simulink library "dspmtrx3"  (Simulink 8.0)
settings: Solver=ode45  SolverMode=SingleTasking  StartTime=0.0  StopTime=10.0  RelTol=1e-3
values from neighbouring files (symbols this model uses):
  a = ver('dsp')    [aboutdspsystbx.m]    (also in dsparch3Transform.m = localGetVal(inData.InstanceData, 'den', '1'); dspddes3Transform.m = sprintf('getYuleWalkerIIRFilterDesignOutput(; dspfdes.m = []; dsprprim.m = a-Mi)
  D = D + B    [rebuffer_delay.m]
undefined symbols (not defined in the file or in its folder): Floor
libraries: dspmtrx3 x5, dspsolvers x3, dspsigattribs x2, dspobslib x1, dspstat3 x1, dspfactors x1
(part 2 of 2)

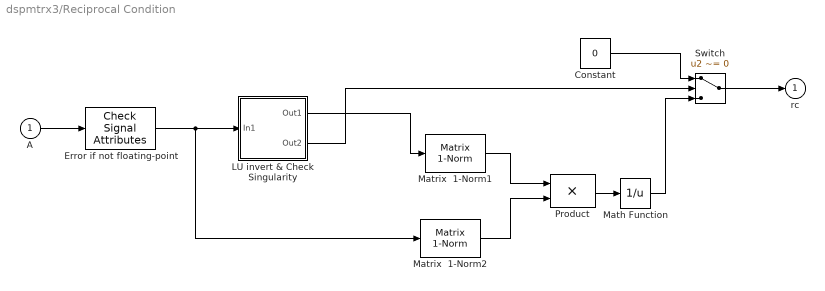
== system dspmtrx3/Reciprocal Condition ==
  A : Inport
  Constant : Constant  Value=0  OutDataTypeStr=Inherit: Inherit via back propagation
  Error if not floating-point : dspsigattribs/Check Signal Attributes  SystemSampleTime=-1  SigAttribCheckMethod=Does not match attributes exactly  Complexity=Ignore  Frame=Ignore  DimsCheckMethod=Ignore  Dimensions=1-D  DatatypeCheckMethod=Is...  DatatypeGeneral=Floating-point  DtypeFloatSpecific=Any floating-point  DtypeFixedSpecific=Any fixed-point  DtypeIntSpecific=Any integer  SampleMode=Ignore
  LU invert & Check Singularity : Subsystem
      mask Display:
      | port_label('output',1,'Inv');
      | port_label('output',2,'Status');
      | port_label('input',1,'Mx');
  Math Function : Math  Operator=reciprocal  SaturateOnIntegerOverflow=on
  Matrix  1-Norm1 : dspmtrx3/Matrix  1-Norm  outputDataTypeStr=Inherit: Same as accumulator  outputLastDataTypeStr=Inherit: Same as accumulator  outputMin=[]  outputMax=[]  roundingMode=Floor  overflowMode=off
  Matrix  1-Norm2 : dspmtrx3/Matrix  1-Norm  outputDataTypeStr=Inherit: Same as accumulator  outputLastDataTypeStr=Inherit: Same as accumulator  outputMin=[]  outputMax=[]  roundingMode=Floor  overflowMode=off
  Product : Product  SaturateOnIntegerOverflow=on  InputSameDT=on  OutDataTypeStr=Inherit: Same as first input
  Switch : Switch  Criteria=u2 ~= 0  InputSameDT=on
  " rc" : Outport  InitialOutput=0
  wires:
  LU invert & Check Singularity/2(Out2) -> Switch/2
  Math Function/1 -> Switch/3
  Switch/1 -> " rc"/1
  Product/1 -> Math Function/1
  Matrix  1-Norm2/1 -> Product/2
  Matrix  1-Norm1/1 -> Product/1
  Constant/1 -> Switch/1
  LU invert & Check Singularity/1(Out1) -> Matrix  1-Norm1/1
  A/1 -> Error if not floating-point/1
  Error if not floating-point/1 -> LU invert & Check Singularity/1(In1), Matrix  1-Norm2/1

== system dspmtrx3/Transpose ==
  In1 : Inport
  Math Function : Math  Operator=transpose  SaturateOnIntegerOverflow=on
  Out1 : Outport
  wires:
  In1/1 -> Math Function/1
  Math Function/1 -> Out1/1

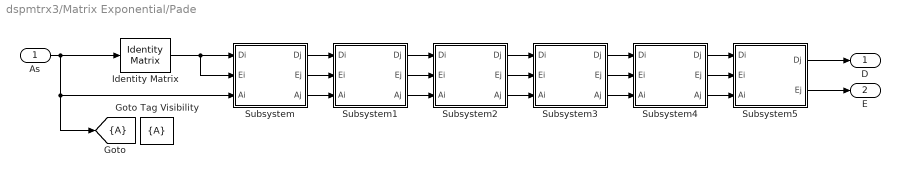
== system dspmtrx3/Matrix Exponential/Pade ==
  As : Inport
  Goto Tag Visibility : GotoTagVisibility
  Identity Matrix : dspmtrx3/Identity Matrix  Inherit=on  N=5  Ts=1  dataType=double  isSigned=on  wordLen=16  udDataType=sfix(16)  fracBitsMode=Best precision  numFracBits=15
  Subsystem : Subsystem
      mask Display: disp('Pade\n1')
  Subsystem1 : Subsystem
      mask Display: disp('Pade\n2')
  Subsystem2 : Subsystem
      mask Display: disp('Pade\n3')
  Subsystem3 : Subsystem
      mask Display: disp('Pade\n4')
  Subsystem4 : Subsystem
      mask Display: disp('Pade\n5')
  Subsystem5 : Subsystem
      mask Display: disp('Pade\n6')
  D : Outport
  E : Outport  Port=2
  tag scope: A=scoped
  wires:
  As/1 -> Identity Matrix/1, Subsystem/3(Ai), [A]
  Identity Matrix/1 -> Subsystem/1(Di), Subsystem/2(Ei)
  Subsystem/1(Dj) -> Subsystem1/1(Di)
  Subsystem/2(Ej) -> Subsystem1/2(Ei)
  Subsystem1/1(Dj) -> Subsystem2/1(Di)
  Subsystem1/2(Ej) -> Subsystem2/2(Ei)
  Subsystem2/1(Dj) -> Subsystem3/1(Di)
  Subsystem2/2(Ej) -> Subsystem3/2(Ei)
  Subsystem3/1(Dj) -> Subsystem4/1(Di)
  Subsystem3/2(Ej) -> Subsystem4/2(Ei)
  Subsystem4/1(Dj) -> Subsystem5/1(Di)
  Subsystem4/2(Ej) -> Subsystem5/2(Ei)
  Subsystem5/2(Ej) -> E/1
  Subsystem5/1(Dj) -> D/1
  Subsystem/3(Aj) -> Subsystem1/3(Ai)
  Subsystem1/3(Aj) -> Subsystem2/3(Ai)
  Subsystem2/3(Aj) -> Subsystem3/3(Ai)
  Subsystem3/3(Aj) -> Subsystem4/3(Ai)
  Subsystem4/3(Aj) -> Subsystem5/3(Ai)

== system dspmtrx3/Matrix Exponential/Scale In ==
  A : Inport
  Inf norm : Subsystem
      mask Display: disp('inf\nnorm')
  Pow2 Scaling : Subsystem
      mask Display: disp('s-scaling')
  Scale Input : Subsystem
  log2 : Subsystem
      mask Display: disp('log2')
  As : Outport
  s : Outport  Port=2
  wires:
  A/1 -> Inf norm/1(In1), Scale Input/2(A)
  Inf norm/1(Out1) -> log2/1(u)
  log2/1(e) -> Pow2 Scaling/1(In1)
  Pow2 Scaling/1(Out1) -> Scale Input/1(s), s/1
  Scale Input/1(sA) -> As/1

== system dspmtrx3/Matrix Exponential/Scale Out ==
  E : Inport
  s : Inport  Port=2
  Frame Conversion : FrameConversion  OutFrame=Sample-based
  Matrix Squaring : Subsystem  TreatAsAtomicUnit=on
  Switch : Switch  Criteria=u2 ~= 0  SaturateOnIntegerOverflow=on
  expm : Outport
  wires:
  s/1 -> Switch/2, Frame Conversion/1
  E/1 -> Matrix Squaring/1(E), Switch/3
  Matrix Squaring/1(Out) -> Switch/1
  Switch/1 -> expm/1
  Frame Conversion/1 -> Matrix Squaring/2(N)

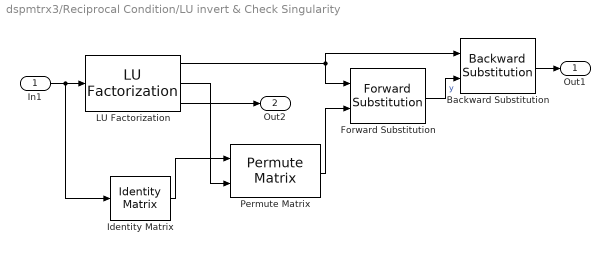
== system dspmtrx3/Reciprocal Condition/LU invert & Check Singularity ==
  In1 : Inport
  Backward Substitution : dspsolvers/Backward Substitution  Unit=off  RealDiag=off  outputMin=[]  outputMax=[]  accumDataTypeStr=Inherit: Same as product output  accumLastDataTypeStr=Inherit: Same as product output  roundingMode=Floor  overflowMode=off
  Forward Substitution : dspsolvers/Forward Substitution  Unit=on  RealDiag=on  outputMin=[]  outputMax=[]  accumDataTypeStr=Inherit: Same as product output  accumLastDataTypeStr=Inherit: Same as product output  roundingMode=Floor  overflowMode=off
  Identity Matrix : dspmtrx3/Identity Matrix  Inherit=on  N=5  Ts=1  dataType=double  isSigned=on  wordLen=16  udDataType=sfix(16)  fracBitsMode=Best precision  numFracBits=15
  LU Factorization : dspfactors/LU Factorization  singular=on  roundingMode=Floor  overflowMode=off
  Permute Matrix : dspmtrx3/Permute Matrix  mode=Rows  ZeroOneIdxMode=One-based  errmode=Clip index  checkDims=on
  Out1 : Outport
  Out2 : Outport  Port=2
  wires:
  LU Factorization/3 -> Out2/1
  LU Factorization/2 -> Permute Matrix/2
  LU Factorization/1 -> Backward Substitution/1, Forward Substitution/1
  Backward Substitution/1 -> Out1/1
  In1/1 -> LU Factorization/1, Identity Matrix/1
  Forward Substitution/1 -> Backward Substitution/2  "y"
  Permute Matrix/1 -> Forward Substitution/2
  Identity Matrix/1 -> Permute Matrix/1

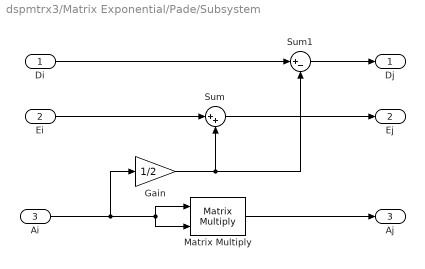
== system dspmtrx3/Matrix Exponential/Pade/Subsystem ==
  Di : Inport
  Ei : Inport  Port=2
  Ai : Inport  Port=3
  Gain : Gain  Gain=1/2  SaturateOnIntegerOverflow=on  OutDataTypeStr=Inherit: Same as input  ParamDataTypeStr=Inherit: Same as input
  Matrix Multiply : Product  Multiplication=Matrix(*)
  Sum : Sum  Inputs=|++  OutDataTypeStr=Inherit: Inherit via back propagation  SaturateOnIntegerOverflow=on
  Sum1 : Sum  Inputs=|+-  OutDataTypeStr=Inherit: Inherit via back propagation  SaturateOnIntegerOverflow=on
  Dj : Outport
  Ej : Outport  Port=2
  Aj : Outport  Port=3
  wires:
  Ei/1 -> Sum/1
  Sum/1 -> Ej/1
  Sum1/1 -> Dj/1
  Di/1 -> Sum1/1
  Gain/1 -> Sum/2, Sum1/2
  Ai/1 -> Gain/1, Matrix Multiply/2, Matrix Multiply/1
  Matrix Multiply/1 -> Aj/1

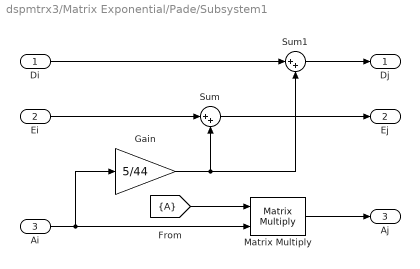
== system dspmtrx3/Matrix Exponential/Pade/Subsystem1 ==
  Di : Inport
  Ei : Inport  Port=2
  Ai : Inport  Port=3
  Gain : Gain  Gain=5/44  OutDataTypeStr=Inherit: Same as input  ParamDataTypeStr=Inherit: Same as input
  Matrix Multiply : Product  Multiplication=Matrix(*)
  Sum : Sum  Inputs=|++  OutDataTypeStr=Inherit: Inherit via back propagation  SaturateOnIntegerOverflow=on
  Sum1 : Sum  Inputs=|++  OutDataTypeStr=Inherit: Inherit via back propagation  SaturateOnIntegerOverflow=on
  Dj : Outport
  Ej : Outport  Port=2
  Aj : Outport  Port=3
  wires:
  Di/1 -> Sum1/1
  Sum1/1 -> Dj/1
  Sum/1 -> Ej/1
  Ei/1 -> Sum/1
  Gain/1 -> Sum/2, Sum1/2
  Ai/1 -> Gain/1, Matrix Multiply/2
  Matrix Multiply/1 -> Aj/1
  [A] -> Matrix Multiply/1

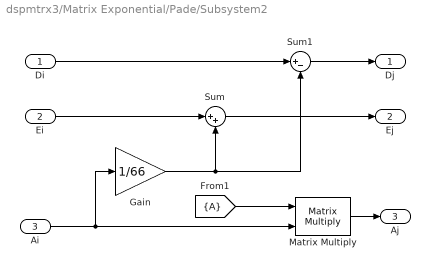
== system dspmtrx3/Matrix Exponential/Pade/Subsystem2 ==
  Di : Inport
  Ei : Inport  Port=2
  Ai : Inport  Port=3
  Gain : Gain  Gain=1/66  OutDataTypeStr=Inherit: Same as input  ParamDataTypeStr=Inherit: Same as input
  Matrix Multiply : Product  Multiplication=Matrix(*)
  Sum : Sum  Inputs=|++  OutDataTypeStr=Inherit: Inherit via back propagation  SaturateOnIntegerOverflow=on
  Sum1 : Sum  Inputs=|+-  OutDataTypeStr=Inherit: Inherit via back propagation  SaturateOnIntegerOverflow=on
  Dj : Outport
  Ej : Outport  Port=2
  Aj : Outport  Port=3
  wires:
  Gain/1 -> Sum1/2, Sum/2
  Di/1 -> Sum1/1
  Sum1/1 -> Dj/1
  Sum/1 -> Ej/1
  Ei/1 -> Sum/1
  Ai/1 -> Matrix Multiply/2, Gain/1
  [A] -> Matrix Multiply/1
  Matrix Multiply/1 -> Aj/1

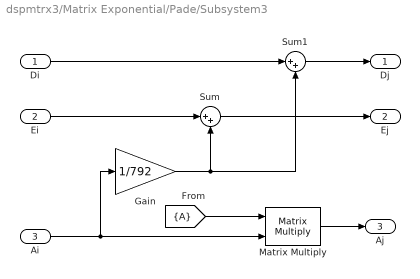
== system dspmtrx3/Matrix Exponential/Pade/Subsystem3 ==
  Di : Inport
  Ei : Inport  Port=2
  Ai : Inport  Port=3
  Gain : Gain  Gain=1/792  OutDataTypeStr=Inherit: Same as input  ParamDataTypeStr=Inherit: Same as input
  Matrix Multiply : Product  Multiplication=Matrix(*)
  Sum : Sum  Inputs=|++  OutDataTypeStr=Inherit: Inherit via back propagation  SaturateOnIntegerOverflow=on
  Sum1 : Sum  Inputs=|++  OutDataTypeStr=Inherit: Inherit via back propagation  SaturateOnIntegerOverflow=on
  Dj : Outport
  Ej : Outport  Port=2
  Aj : Outport  Port=3
  wires:
  Gain/1 -> Sum1/2, Sum/2
  Ei/1 -> Sum/1
  Sum/1 -> Ej/1
  Sum1/1 -> Dj/1
  Di/1 -> Sum1/1
  Ai/1 -> Matrix Multiply/2, Gain/1
  Matrix Multiply/1 -> Aj/1
  [A] -> Matrix Multiply/1

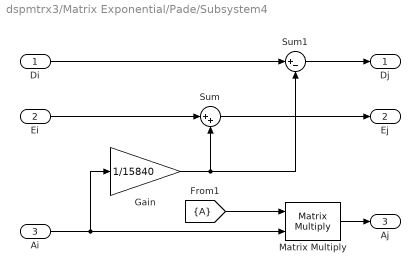
== system dspmtrx3/Matrix Exponential/Pade/Subsystem4 ==
  Di : Inport
  Ei : Inport  Port=2
  Ai : Inport  Port=3
  Gain : Gain  Gain=1/15840  OutDataTypeStr=Inherit: Same as input  ParamDataTypeStr=Inherit: Same as input
  Matrix Multiply : Product  Multiplication=Matrix(*)
  Sum : Sum  Inputs=|++  OutDataTypeStr=Inherit: Inherit via back propagation  SaturateOnIntegerOverflow=on
  Sum1 : Sum  Inputs=|+-  OutDataTypeStr=Inherit: Inherit via back propagation  SaturateOnIntegerOverflow=on
  Dj : Outport
  Ej : Outport  Port=2
  Aj : Outport  Port=3
  wires:
  Ei/1 -> Sum/1
  Sum/1 -> Ej/1
  Sum1/1 -> Dj/1
  Di/1 -> Sum1/1
  Gain/1 -> Sum/2, Sum1/2
  Ai/1 -> Matrix Multiply/2, Gain/1
  [A] -> Matrix Multiply/1
  Matrix Multiply/1 -> Aj/1

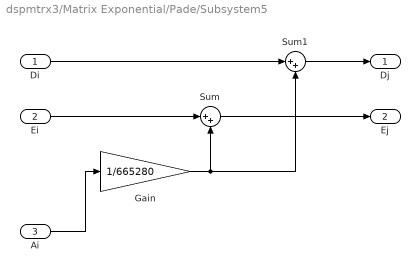
== system dspmtrx3/Matrix Exponential/Pade/Subsystem5 ==
  Di : Inport
  Ei : Inport  Port=2
  Ai : Inport  Port=3
  Gain : Gain  Gain=1/665280  OutDataTypeStr=Inherit: Same as input  ParamDataTypeStr=Inherit: Same as input
  Sum : Sum  Inputs=|++  OutDataTypeStr=Inherit: Inherit via back propagation  SaturateOnIntegerOverflow=on
  Sum1 : Sum  Inputs=|++  OutDataTypeStr=Inherit: Inherit via back propagation  SaturateOnIntegerOverflow=on
  Dj : Outport
  Ej : Outport  Port=2
  wires:
  Di/1 -> Sum1/1
  Sum1/1 -> Dj/1
  Sum/1 -> Ej/1
  Ei/1 -> Sum/1
  Gain/1 -> Sum/2, Sum1/2
  Ai/1 -> Gain/1

== system dspmtrx3/Matrix Exponential/Scale In/Inf norm ==
  In1 : Inport
  Abs : Abs  SaturateOnIntegerOverflow=on
  Math Function : Math  Operator=conj  SaturateOnIntegerOverflow=on
  Matrix Sum : dspobslib/Matrix Sum  Dim=Rows  roundingMode=Floor  overflowMode=off
  Maximum : dspstat3/Maximum  fcn=Value  reset=None  indexBase=One  operateOver=Each column  Dimension=1  colComp=on  operation=maximum  roiEnable=off  roiType=Rectangles  roiPortion=Entire ROI  roiOutput=Individual statistics for each ROI  roiFlag=off  roundingMode=Floor  overflowMode=off
  Out1 : Outport
  wires:
  Matrix Sum/1 -> Abs/1
  In1/1 -> Math Function/1
  Maximum/1 -> Out1/1
  Math Function/1 -> Matrix Sum/1
  Abs/1 -> Maximum/1

== system dspmtrx3/Matrix Exponential/Scale In/Pow2 Scaling ==
  In1 : Inport
  Constant : Constant  Value=0  VectorParams1D=off  OutDataTypeStr=int32
  Constant1 : Constant  VectorParams1D=off  OutDataTypeStr=int32
  MinMax : MinMax  Function=max  Inputs=2  SaturateOnIntegerOverflow=on  InputSameDT=on
  Sum : Sum  Inputs=++|  SaturateOnIntegerOverflow=on
  Out1 : Outport
  wires:
  Sum/1 -> MinMax/1
  Constant/1 -> MinMax/2
  In1/1 -> Sum/2
  MinMax/1 -> Out1/1
  Constant1/1 -> Sum/1

== system dspmtrx3/Matrix Exponential/Scale In/Scale Input ==
  s : Inport
  A : Inport  Port=2
  Data Type Conversion : DataTypeConversion  SaturateOnIntegerOverflow=on  RndMeth=Zero
  Math Function : Math  Operator=reciprocal  SaturateOnIntegerOverflow=on
  Product : Product  SaturateOnIntegerOverflow=on  OutDataTypeStr=Inherit: Same as first input
  Two^N : Subsystem
      mask Display: disp('2.^N')
  sA : Outport
  wires:
  Two^N/1(Out) -> Data Type Conversion/1
  Data Type Conversion/1 -> Math Function/1
  s/1 -> Two^N/1(N)
  Product/1 -> sA/1
  Math Function/1 -> Product/2
  A/1 -> Product/1

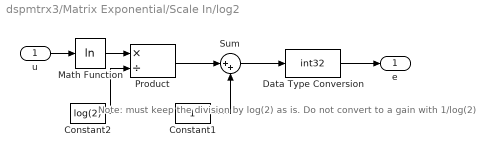
== system dspmtrx3/Matrix Exponential/Scale In/log2 ==
  note: Note: must keep the division
      | by log(2) as is.  Do not convert
      | to a gain with 1/log(2)
  u : Inport
  Constant1 : Constant  VectorParams1D=off  OutDataTypeStr=Inherit: Inherit via back propagation
  Constant2 : Constant  Value=log(2)  VectorParams1D=off  OutDataTypeStr=Inherit: Inherit via back propagation
  Data Type Conversion : DataTypeConversion  OutDataTypeStr=int32  SaturateOnIntegerOverflow=on  RndMeth=Zero
  Math Function : Math  Operator=log  SaturateOnIntegerOverflow=on
  Product : Product  Inputs=*/  SaturateOnIntegerOverflow=on  OutDataTypeStr=Inherit: Same as first input
  Sum : Sum  Inputs=|++  OutDataTypeStr=Inherit: Inherit via back propagation  RndMeth=Ceiling
  e : Outport
  wires:
  Constant2/1 -> Product/2
  Math Function/1 -> Product/1
  u/1 -> Math Function/1
  Data Type Conversion/1 -> e/1
  Product/1 -> Sum/1
  Sum/1 -> Data Type Conversion/1
  Constant1/1 -> Sum/2

== system dspmtrx3/Matrix Exponential/Scale Out/Matrix Squaring ==
  E : Inport
  N : Inport  Port=2
  For Iterator : ForIterator  ResetStates=reset  IterationSource=external
  Matrix Multiply : Product  Multiplication=Matrix(*)
  Switch : Switch  Criteria=u2 > Threshold  Threshold=1  SaturateOnIntegerOverflow=on
  Unit Delay : UnitDelay  SampleTime=-1
  Out : Outport
  wires:
  N/1 -> For Iterator/1
  E/1 -> Switch/3
  For Iterator/1 -> Switch/2
  Unit Delay/1 -> Switch/1
  Matrix Multiply/1 -> Unit Delay/1, Out/1
  Switch/1 -> Matrix Multiply/1, Matrix Multiply/2

== system dspmtrx3/Matrix Exponential/Scale In/Scale Input/Two^N ==
  note: Compensate
      | for 1-based loops
  N : Inport
  2^N : Subsystem  TreatAsAtomicUnit=on
  Constant : Constant  VectorParams1D=off  OutDataTypeStr=Inherit: Inherit via back propagation
  Frame Conversion : FrameConversion  OutFrame=Sample-based
  Sum : Sum  Inputs=|++  SaturateOnIntegerOverflow=on
  Out : Outport
  wires:
  Constant/1 -> Sum/2
  Sum/1 -> Frame Conversion/1
  N/1 -> Sum/1
  2^N/1(Out) -> Out/1
  Frame Conversion/1 -> 2^N/1(N)

== system dspmtrx3/Matrix Exponential/Scale In/Scale Input/Two^N/2^N ==
  N : Inport
  Bitwise Logical Operator2 : ArithShift  BitShiftNumber=-(1)
  For Iterator : ForIterator  ResetStates=reset  IterationSource=external  ShowIterationPort=off
  Signal Specification : SignalSpecification  OutDataTypeStr=uint32
  Unit Delay : UnitDelay  X0=uint32(1)  SampleTime=-1
  Out : Outport
  wires:
  N/1 -> For Iterator/1
  Unit Delay/1 -> Out/1, Signal Specification/1
  Bitwise Logical Operator2/1 -> Unit Delay/1
  Signal Specification/1 -> Bitwise Logical Operator2/1
